simulink subsystem "srp_acceleration"  (R2023b)
settings: Solver=VariableStepAuto  StartTime=0.0  StopTime=10.0  RelTol=1e-3
model mask{earth_radius=0, sun_radius=0, moon_radius=0, A_sc=0, m_sc=0, AU=0, P=0}
  mask prompts: earth_radius "Earth radius"; sun_radius "Sun radius"; moon_radius "Moon radius"; A_sc "Spacecraft Area"; m_sc "Spacecraft Mass"; AU "Astronomical Unit conversion"; P "Radiation pressure"
libraries: dyn_lib x4
settings Model: Creator=brent  LastModifiedBy=brent

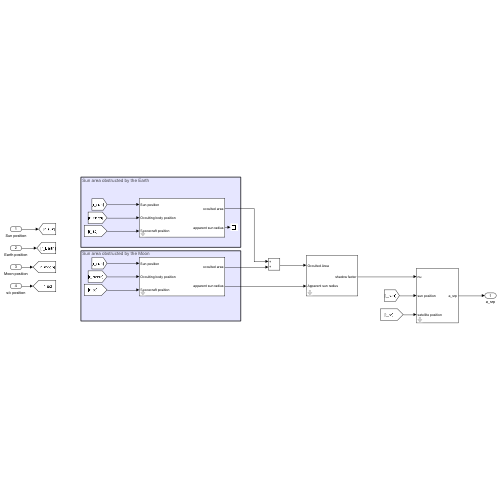
[thumbnail: Simulink's stored preview of the top-level diagram]
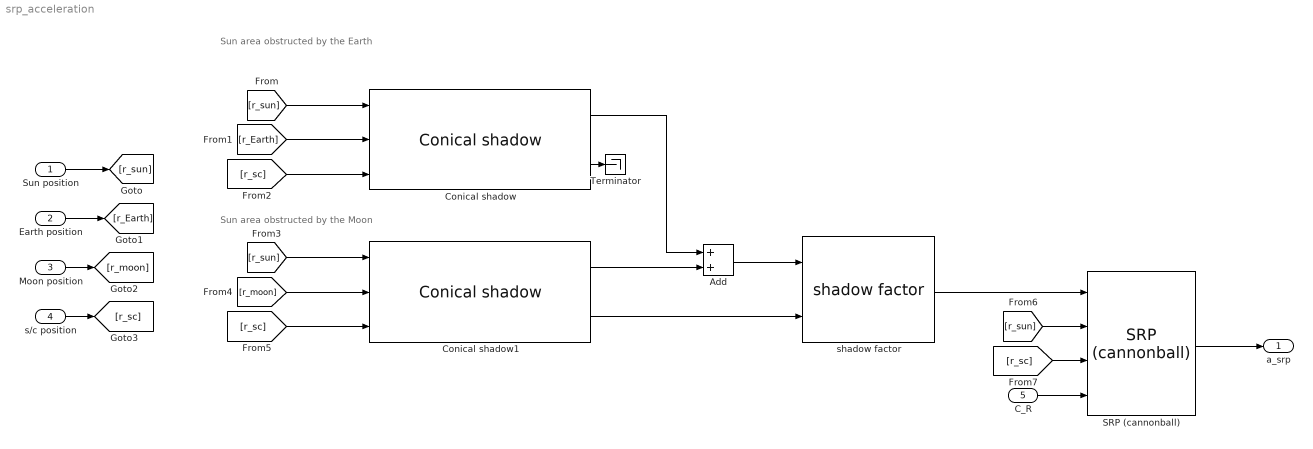
== system srp_acceleration ==
  note: Sun area obstructed by the Earth
  note: Sun area obstructed by the Moon
  Sun position : Inport
  Earth position : Inport  Port=2
  Moon position : Inport  Port=3
  s/c position : Inport  Port=4
  C_R : Inport  Port=5
  Add : Sum  InputSameDT=on  SaturateOnIntegerOverflow=on
  Conical shadow : dyn_lib/Conical shadow  R_B=earth_radius  R_S=sun_radius
      settings: SourceProductName=Dynamics library
  Conical shadow1 : dyn_lib/Conical shadow  R_B=moon_radius  R_S=sun_radius
      settings: SourceProductName=Dynamics library
  SRP (cannonball) : dyn_lib/SRP (cannonball)  A_sc=A_sc  m=m_sc  AU=AU  P=P
      settings: SourceProductName=Dynamics library
  Terminator : Terminator
  shadow factor : dyn_lib/shadow factor
      settings: SourceProductName=Dynamics library
  a_srp : Outport
  wires:
  shadow factor/1 -> SRP (cannonball)/1
  [r_sc] -> SRP (cannonball)/3
  [r_sun] -> SRP (cannonball)/2
  Add/1 -> shadow factor/1
  Conical shadow/1 -> Add/1
  Conical shadow1/1 -> Add/2
  Conical shadow1/2 -> shadow factor/2
  Conical shadow/2 -> Terminator/1
  [r_moon] -> Conical shadow1/2
  [r_sc] -> Conical shadow1/3
  [r_sun] -> Conical shadow1/1
  [r_sc] -> Conical shadow/3
  [r_Earth] -> Conical shadow/2
  [r_sun] -> Conical shadow/1
  s/c position/1 -> [r_sc]
  Moon position/1 -> [r_moon]
  Earth position/1 -> [r_Earth]
  Sun position/1 -> [r_sun]
  SRP (cannonball)/1 -> a_srp/1
  C_R/1 -> SRP (cannonball)/4
